simulink model "plant"  (R2025b)
settings: Solver=VariableStepAuto  StartTime=0.0  StopTime=0.001  RelTol=1e-3
values from neighbouring files (symbols this model uses):
  tau = 5    [plant_coeffs.m]
undefined symbols (not defined in the file or in its folder): Rows
libraries: dspsigops x1
settings Model: Creator=strog  LastModifiedBy=strog

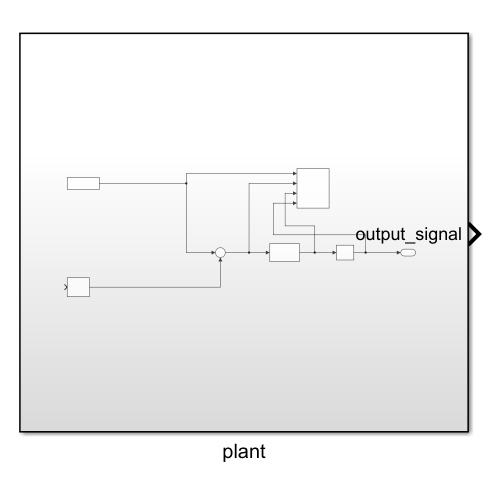
[thumbnail: Simulink's stored preview of the top-level diagram]
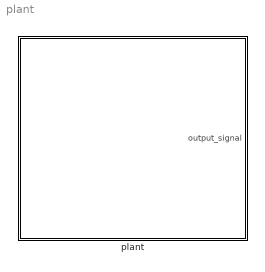
== system plant ==
  plant : Subsystem

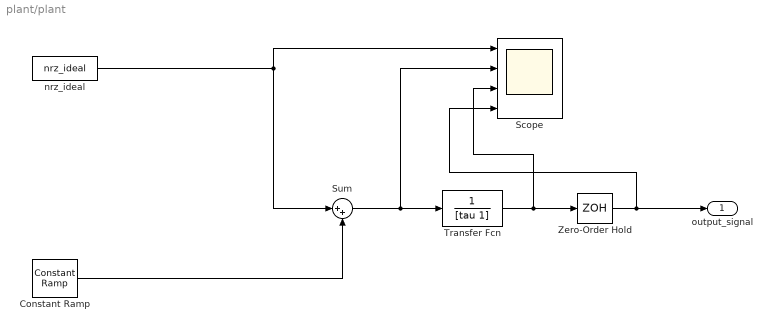
== system plant/plant ==
  Constant Ramp : dspsigops/Constant Ramp  L=Rows  dim=1  Slope=0.001  dataType=Same as input  isSigned=on  wordLen=16  udDataType=sfix(16)  fracBitsMode=Best precision  numFracBits=15  Offset=0
  Scope : Scope  NumInputPorts=4
      settings: ActiveDisplayYMinimum=-8.4177738313956336  ActiveDisplayYMaximum=12.220378904493744  DataLoggingVariableName=ScopeData2  DataLoggingSaveFormat=Array
  Sum : Sum  Inputs=|++
  Transfer Fcn : TransferFcn  Denominator=[tau 1]
  Zero-Order Hold : ZeroOrderHold  SampleTime=0.01
  nrz_ideal : FromWorkspace  VariableName=nrz_ideal  OutDataTypeStr=double  SampleTime=1/8192000
  output_signal : Outport
  wires:
  Zero-Order Hold/1 -> Scope/4, output_signal/1
  Sum/1 -> Scope/2, Transfer Fcn/1
  Transfer Fcn/1 -> Scope/3, Zero-Order Hold/1
  nrz_ideal/1 -> Sum/1, Scope/1
  Constant Ramp/1 -> Sum/2
